simulink model "linearized_smm_with_lqr_2d"  (R2014b)
settings: Solver=FixedStepDiscrete  StartTime=0.0  StopTime=inf  FixedStep=sample_time  RelTol=1e-3
undefined symbols (not defined in the file): A_kalman_fourbar_gear, A_kalman_transverse, A_kalman_vertical, A_lpf_dtau, A_lpf_leg_spring, B1_lpf_dtau, B1_lpf_leg_spring, B2_lpf_dtau, B2_lpf_leg_spring, B_dx_versus_x0, B_kalman_fourbar_gear, B_kalman_transverse, B_kalman_vertical, backwards_K_sag_of_t, boom_mount_angle, C_kalman_fourbar_gear, C_kalman_transverse, C_kalman_vertical, com_leg_motor, com_torso, contact_threshold, control_start_time, d_vertical_boom_com_offset, d_vertical_com, desired_com_apex_height, desired_com_forward_velocity, desired_torso_angle, Discrete, fcut_contact, forward_dx, forward_dx_of_dxstar, forward_x, forward_x_of_dxstar, g, h_boom, HIP_MTR_MAX_CONT_TORQUE, i_robot, initial_dx_estimate, initial_dy_estimate, initial_dz_estimate, initial_z_estimate, j_leg, j_motor, j_segments, k_LQR_vertical, k_sea, k_vertical_winch, kalman_load_to_deflect_transmission, kalman_stance_slip_threshold, kd_lateral, kd_motor, kp_lateral, kp_motor, l_boom_projected, l_retract_delta, l_retract_swing_max, l_retract_swing_min, l_seg, lambda1, lambda2 ... (+60)
libraries: simulink x14, ctrlSharedLib x7
(part 4 of 4)

== matlab function linearized_smm_with_lqr_2d/Control/Behavior Control/Primary Leg Behavior/Running/Closed Loop Compensation/ESTIMATE CLOSED LOOP ERROR X FOR VARIABLE SPEED ==
  data: dx_land_hist input; A_cl output; delta_ux_hist input; dx_lift_hist input; dx_star_hist input; B_dx_versus_x0 parameter; W_real input; epsilon_0 output; c output; A_cl_nb output; epsilon_0_nb output; c_nb output
function [A_cl, epsilon_0, c, ...
          A_cl_nb, epsilon_0_nb, c_nb] = error_fitting_dxstar...
         (dx_land_hist, delta_ux_hist, dx_lift_hist, dx_star_hist,...
          B_dx_versus_x0, W_real)
% data_length = min([length(dx_lift_hist), filter_length]);
data_length = length(dx_lift_hist);
assert(data_length < 100);
% add fake data
fake_dx_land_err_magnitude = 0.1; fake_dx_star_magnitude = 0.1;
[fgrid_dx_land_err, fgrid_dx_star, fgrid_dx_lift_err] = ...
    meshgrid(fake_dx_land_err_magnitude*[-1 1],fake_dx_star_magnitude*[-1 1],0);
fake_data_length = numel(fgrid_dx_land_err);
fake_dx_land_err = fgrid_dx_land_err(:);
fake_dx_star = fgrid_dx_star(:);
fake_dx_lift_err = fgrid_dx_lift_err(:);
fake_delta_ux = zeros(fake_data_length,1);
% assert(fake_data_length<100);
% assert(filter_length<100);
% fake_dx_land_err = linspace(-0.1, 0.1, fake_data_length)';
% fake_dx_lift_err = zeros(fake_data_length,1);
% fake_delta_ux = zeros(fake_data_length,1);
% fake_dx_star = linspace(-0.25, 0.25, fake_data_length)';
dx_land_err = [reshape(dx_land_hist(1:data_length)-dx_star_hist(1:data_length),...
                       data_length, 1); fake_dx_land_err];
dx_lift_err = [reshape(dx_lift_hist(1:data_length)-dx_star_hist(1:data_length),...
                       data_length, 1); fake_dx_lift_err];
dx_star = [reshape(dx_star_hist(1:data_length), data_length,1); fake_dx_star];
delta_ux = [reshape(delta_ux_hist(1:data_length), data_length, 1); fake_delta_ux];
% weighted least squares
W = diag([W_real*ones(1,data_length), ones(1,fake_data_length)]);
Y = dx_lift_err - B_dx_versus_x0*delta_ux;
X = [dx_land_err, dx_star, ones(data_length+fake_data_length,1)];
% linear regression for s_{i+1}-s0 = A_cl*(s_i-s0) + epsilon_0 + c(s0) + B*delta_u
% solve for Y = X*beta, beta column vector
beta_hat = (X'*W*X)\X'*W*Y;
W_nobias = diag([W_real*ones(1,data_length), 0.001*ones(1,fake_data_length)]);
beta_hat_nobias = (X'*W_nobias*X)\X'*W_nobias*Y;
A_cl = beta_hat(1);
c = beta_hat(2);
epsilon_0 = beta_hat(3);
A_cl_nb = beta_hat_nobias(1);
c_nb = beta_hat_nobias(2);
epsilon_0_nb = beta_hat_nobias(3);

== matlab function linearized_smm_with_lqr_2d/Control/Behavior Control/Primary Leg Behavior/Running/Closed Loop Compensation/CLOSED LOOP COMPENSATION Y FOR VAIRABLE SPEED ==
  data: A_cl input; epsilon input; c input; delta_s_i input; dx_star input; B_cl input; delta_ux output
function delta_ux  = closed_loop_compensation_dxstar...
         (A_cl,epsilon, c, delta_s_i, dx_star, B_cl)
% assume form of delta_s_{i+1} = A_cl*delta_s_i + epsilon +c*dx_star + B_cl*delta_ux
% where delta measures deviation from deadbeat case. solve for
% delta_ux = (-A_cl*delta_s_i-epsilon - c*dxstar)/B_cl to achieve deadbeat
delta_ux = (-A_cl*delta_s_i - epsilon - c*dx_star)/B_cl;

== matlab function linearized_smm_with_lqr_2d/Control/Behavior Control/Primary Secondary Leg Swap/ToggleRightLeftLeg ==
  data: toggle input boolean; right_left output double; previous_right_left input double
function right_left = ToggleRightLeftLeg(toggle, previous_right_left)
    
    if toggle
        right_left = -previous_right_left + 1;
    else
        right_left = previous_right_left;
    end

end

== matlab function linearized_smm_with_lqr_2d/Control/Behavior Control/Lateral Control ==
  data: hopping input; right_left input; tau_r output size=1; qLateralR input; dqLateralR input; qLateralL input; dqLateralL input; F_leg_R input; F_leg_L input; deadbeat_enabled input; target_primary_deadbeat_angle input; lateral_transition_force parameter; lateral_target_angle_right parameter; m_leg_motor parameter; m_leg parameter; m_total_real parameter; g parameter; lateral_offset parameter; tau_l output size=1; kp_lateral parameter; kd_lateral parameter; minimum_lateral_angle parameter; maximum_lateral_angle parameter; HIP_MTR_MAX_CONT_TORQUE parameter; torso_centerline_roll_offset_angle parameter
function [tau_r, tau_l] = LateralBoomControl(hopping, right_left, qLateralR, dqLateralR, qLateralL, dqLateralL, F_leg_R, F_leg_L, deadbeat_enabled, target_primary_deadbeat_angle, lateral_transition_force, lateral_target_angle_right, m_leg_motor, m_leg, m_total_real, g, lateral_offset, kp_lateral, kd_lateral, minimum_lateral_angle, maximum_lateral_angle, HIP_MTR_MAX_CONT_TORQUE, torso_centerline_roll_offset_angle)
    
    % Only add gravity compensation to PD when suspended from winch (approximately static)
    gravity_compensation = 0;
    if ~hopping, gravity_compensation = (m_leg_motor+m_leg)*g*lateral_offset; end
    
    % Inertia for feedforward accelerations
    motor_inertia = (m_leg_motor+m_leg)*lateral_offset^2;
    
    % Right Leg
    right_target = [lateral_target_angle_right, 0, 0];
    if deadbeat_enabled && right_left
        right_target = [pi/2 - target_primary_deadbeat_angle(1) - torso_centerline_roll_offset_angle, -target_primary_deadbeat_angle(2), -target_primary_deadbeat_angle(2)];
    end
    desired = [saturate(right_target(1),minimum_lateral_angle,maximum_lateral_angle), right_target(2)];
    measured = [qLateralR, dqLateralR];
    tau_r = [kp_lateral, kd_lateral] * (desired-measured)' + gravity_compensation + motor_inertia*right_target(3);
    tau_r = max(min(HIP_MTR_MAX_CONT_TORQUE, tau_r),-HIP_MTR_MAX_CONT_TORQUE);
    
    if (F_leg_R >= lateral_transition_force)
        if hopping
            tau_r = -F_leg_R*lateral_offset*(m_total_real-(m_leg_motor+m_leg))/m_total_real;
        else
            tau_r = -lateral_offset*(F_leg_R-(m_leg_motor+m_leg)*g);
        end
    end
    
    % Left Leg
    left_target = [lateral_target_angle_right, 0, 0];
    if deadbeat_enabled && ~right_left
        left_target = [pi/2 - target_primary_deadbeat_angle(1) + torso_centerline_roll_offset_angle, -target_primary_deadbeat_angle(2), -target_primary_deadbeat_angle(2)];
    end
    desired = [saturate(left_target(1),minimum_lateral_angle,maximum_lateral_angle), left_target(2)];
    measured = [qLateralL, dqLateralL];
    tau_l = [kp_lateral, kd_lateral] * (desired-measured)' + gravity_compensation + motor_inertia*left_target(3);
    tau_l = max(min(HIP_MTR_MAX_CONT_TORQUE, tau_l),-HIP_MTR_MAX_CONT_TORQUE);
    
    if (F_leg_L >= lateral_transition_force)
        if hopping
            tau_l = -F_leg_L*lateral_offset*(m_total_real-(m_leg_motor+m_leg))/m_total_real;
        else
            tau_l = -lateral_offset*(F_leg_L-(m_leg_motor+m_leg)*g);
        end
    end
end

function [desired_saturated] = saturate(desired, minimum_lateral_angle, maximum_lateral_angle)
    desired_saturated = desired;
    if desired(1) < minimum_lateral_angle
        desired_saturated = [minimum_lateral_angle, 0];
    elseif desired(1) > maximum_lateral_angle
        desired_saturated = [maximum_lateral_angle, 0];    
    end
end

== matlab function linearized_smm_with_lqr_2d/Control/Behavior Control/Primary Leg Behavior/Running/Stance/Inverse Dynamics 2D/target_GRF_inverse_dynamics ==
  data: GRFx input; GRFz input; right_left input; z output; theta input; phi input; l_leg input; w input; tau_rotor_f input; tau_rotor_b input; d_vertical_com parameter; LEG_MTR_GEAR_RATIO parameter; g parameter; j_leg parameter; i_robot parameter; m_total_real parameter; m_leg parameter
%% Inverse dynamics
% Inputs:  gamma, dgamma, theta, dtheta,  GRFx_des, GRFy_des
% Outputs: ddx,   ddy,    ddl,   ddgamma, ddtheta,  tau_sf,  tau_sb
function z = fcn(GRFx, GRFz, right_left, theta, phi, l_leg, w,...
                                  tau_rotor_f, tau_rotor_b, ...
                                  d_vertical_com, LEG_MTR_GEAR_RATIO, g,...
                                  j_leg, i_robot, ...
                                  m_total_real, m_leg)

              
              
    % Parameters
    m      = m_total_real;    % mass of system + boom
    Il     = j_leg;             % inertia of leg
    It     = i_robot;           % inertia of system3.
    d      = d_vertical_com;             % distance from hip to system COM
    g1     = phi(1)+theta(1);   % global leg angle (after spring)
    dg1    = phi(2)+theta(2);
    th     = theta(1);          % global torso angle   
    dth    = theta(2);
    t_rf   = tau_rotor_f;       % torque applied at front rotor 
    t_rb   = tau_rotor_b;       % torque applied at back rotor
    N      = -LEG_MTR_GEAR_RATIO;
    l      = l_leg(1);          % leg length
    dl     = l_leg(2);
    
    % Stance dynamics (P z = [h; -dJ*dq] + [J zeros(2,2)]^T F)
    %     J  = [1  0  sin(g1)     l*cos(g1)   -d*cos(th);
    %           0  1  cos(g1)    -l*sin(g1)    d*sin(th)];
    %       
    %     dJ = [0  0   dg1*cos(g1)    (-l*dg1*sin(g1)+dl*cos(g1))  d*dth*sin(th);
    %           0  0  -dg1*sin(g1)    (-1*dg1*cos(g1)-dl*sin(g1))  d*dth*cos(th)];
    % 
    %     dq  = [dx  dz  dl  dg1  dth ]';
    %       
    %     M = [m  0   0       0    0; 
    %          0  m   0       0    0;
    %          0  0   m_leg   0    0;   
    %          0  0   0       Il   0;  
    %          0  0   0       0    It];  
    %     
    %     h = [0; -m*g_reduced; 0; 0; (-t_rf-t_rb)];
    % 
    %     S = [ 0         0;
    %           0         0;
    %           1/w      -1/w;
    %           1         1;
    %          -(N-1)/N  -(N-1)/N];
    % 
    %     F = [GRFx GRFz]';
    %     
    %     P = [M              -S;       
    %          J               zeros(2,2)];
    
    % Solving for z:    
    %     ddq = [ddx ddy ddl ddg1 ddth]';
    %     z = [ddq; t_sf; t_sb];
    %     z = P\([h; -dJ*dq] + [J zeros(2,2)]'*F);
    
    z =  [GRFx/m;
         (GRFz - g*m)/m;
        -(Il*d*dg1^2*m*cos(g1 - th) - 2*GRFx*Il*d*sin(th) - 2*Il*d^2*dth^2*m - GRFz*d*l^2*m*cos(th) - GRFx*d*l^2*m*sin(th) - 2*GRFz*Il*d*cos(th) + 2*GRFz*It*N*l*cos(g1) + 2*GRFz*Il*N*d*cos(th) + 2*GRFx*It*N*l*sin(g1) + 2*GRFx*Il*N*d*sin(th) - It*N*dg1^2*l*m + GRFz*d*l^2*m*cos(2*g1 - th) + GRFx*d*l^2*m*sin(2*g1 - th) + 2*Il*d*g*m*cos(th) + Il*d*dg1^2*m*cos(g1 + th) + 2*Il*N*d^2*dth^2*m - It*N*dg1^2*l^2*m - 2*It*N*g*l*m*cos(g1) - 2*Il*N*d*g*m*cos(th) + It*N*dg1^2*l^2*m*cos(2*g1) - Il*N*d*dg1^2*m*cos(g1 + th) - Il*d*dg1^2*l*m*cos(g1 + th) + 4*Il*d*dg1*dl*m*sin(g1 - th) + GRFz*N*d^2*l*m*cos(g1) + GRFz*N*d*l^2*m*cos(th) + GRFx*N*d^2*l*m*sin(g1) + 2*N*d*l*m*t_rb*sin(g1 - th) + 2*N*d*l*m*t_rf*sin(g1 - th) + GRFx*N*d*l^2*m*sin(th) - Il*N*d*dg1^2*m*cos(g1 - th) - GRFz*N*d^2*l*m*cos(g1 - 2*th) + GRFx*N*d^2*l*m*sin(g1 - 2*th) + Il*d*dg1^2*l*m*cos(g1 - th) - It*N*dg1^2*l*m*cos(2*g1) - GRFz*N*d*l^2*m*cos(2*g1 - th) - GRFx*N*d*l^2*m*sin(2*g1 - th) + Il*N*d*dg1^2*l*m*cos(g1 + th) - 4*Il*N*d*dg1*dl*m*sin(g1 - th) - Il*N*d*dg1^2*l*m*cos(g1 - th) + 2*It*N*d*dth^2*l*m*cos(g1 - th))/(2*m*(It*N*l - Il*d*cos(g1 - th) + Il*N*d*cos(g1 - th)));
        -(2*GRFx*It*N*cos(g1) - 2*GRFz*It*N*sin(g1) + GRFx*N*d^2*m*cos(g1 - 2*th) + 4*It*N*dg1*dl*m + GRFz*N*d^2*m*sin(g1 - 2*th) + GRFx*d*l*m*cos(2*g1 - th) - GRFz*d*l*m*sin(2*g1 - th) + It*N*dg1^2*m*sin(2*g1) + 2*It*N*g*m*sin(g1) + GRFx*d*l*m*cos(th) - GRFz*d*l*m*sin(th) + GRFx*N*d^2*m*cos(g1) + 2*N*d*m*t_rb*cos(g1 - th) + 2*N*d*m*t_rf*cos(g1 - th) - GRFz*N*d^2*m*sin(g1) - GRFx*N*d*l*m*cos(th) + GRFz*N*d*l*m*sin(th) - GRFx*N*d*l*m*cos(2*g1 - th) - 2*It*N*d*dth^2*m*sin(g1 - th) + GRFz*N*d*l*m*sin(2*g1 - th) - It*N*dg1^2*l*m*sin(2*g1))/(2*m*(It*N*l - Il*d*cos(g1 - th) + Il*N*d*cos(g1 - th)));
        -(GRFx*Il*cos(g1) - GRFz*Il*sin(g1) - GRFx*Il*N*cos(g1) + (Il*dg1^2*m*sin(2*g1))/2 + GRFz*Il*N*sin(g1) + Il*g*m*sin(g1) + GRFx*l^2*m*cos(g1) - GRFz*l^2*m*sin(g1) + 2*Il*dg1*dl*m + N*l*m*t_rb + N*l*m*t_rf + GRFz*N*l^2*m*sin(g1) - 2*Il*N*dg1*dl*m - Il*d*dth^2*m*sin(g1 - th) - (Il*N*dg1^2*m*sin(2*g1))/2 - (Il*dg1^2*l*m*sin(2*g1))/2 - Il*N*g*m*sin(g1) - GRFx*N*l^2*m*cos(g1) + GRFx*N*d*l*m*cos(th) - GRFz*N*d*l*m*sin(th) + Il*N*d*dth^2*m*sin(g1 - th) + (Il*N*dg1^2*l*m*sin(2*g1))/2)/(m*(It*N*l - Il*d*cos(g1 - th) + Il*N*d*cos(g1 - th)));
        -(2*GRFx*Il*It*N*cos(g1) - 2*GRFz*Il*It*N*sin(g1) - GRFz*Il*d*m*w*cos(th) - 2*GRFz*Il*d*m_leg*w*cos(th) - GRFx*Il*d*m*w*sin(th) - 2*GRFx*Il*d*m_leg*w*sin(th) + GRFx*Il*N*d^2*m*cos(g1) + 2*Il*N*d*m*t_rb*cos(g1 - th) + 2*Il*N*d*m*t_rf*cos(g1 - th) + 2*GRFx*It*N*l^2*m*cos(g1) - GRFz*Il*N*d^2*m*sin(g1) - 2*GRFz*It*N*l^2*m*sin(g1) + GRFx*Il*N*d^2*m*cos(g1 - 2*th) + 4*Il*It*N*dg1*dl*m + GRFz*Il*N*d^2*m*sin(g1 - 2*th) - 2*Il*d^2*dth^2*m*m_leg*w - GRFz*Il*d*m*w*cos(2*g1 - th) - GRFx*Il*d*m*w*sin(2*g1 - th) + Il*It*N*dg1^2*m*sin(2*g1) + 2*Il*It*N*g*m*sin(g1) - GRFx*d*l^2*m*m_leg*w*sin(th) - Il*It*N*dg1^2*l*m*sin(2*g1) + Il*d*dg1^2*m*m_leg*w*cos(g1 - th) + 2*GRFz*It*N*l*m*w*cos(g1) + 2*GRFz*It*N*l*m_leg*w*cos(g1) + GRFz*Il*N*d*m*w*cos(th) + 2*GRFz*Il*N*d*m_leg*w*cos(th) + 2*GRFx*It*N*l*m*w*sin(g1) + 2*GRFx*It*N*l*m_leg*w*sin(g1) + GRFx*Il*N*d*m*w*sin(th) + 2*GRFx*Il*N*d*m_leg*w*sin(th) - It*N*dg1^2*l*m*m_leg*w + GRFz*d*l^2*m*m_leg*w*cos(2*g1 - th) + GRFx*d*l^2*m*m_leg*w*sin(2*g1 - th) + 2*Il*d*g*m*m_leg*w*cos(th) + Il*d*dg1^2*m*m_leg*w*cos(g1 + th) + 2*Il*N*d^2*dth^2*m*m_leg*w - It*N*dg1^2*l^2*m*m_leg*w - 2*Il*It*N*d*dth^2*m*sin(g1 - th) + GRFz*Il*N*d*m*w*cos(2*g1 - th) + GRFx*Il*N*d*m*w*sin(2*g1 - th) - GRFz*d*l^2*m*m_leg*w*cos(th) + It*N*dg1^2*l^2*m*m_leg*w*cos(2*g1) - Il*N*d*dg1^2*m*m_leg*w*cos(g1 + th) - Il*d*dg1^2*l*m*m_leg*w*cos(g1 + th) + 4*Il*d*dg1*dl*m*m_leg*w*sin(g1 - th) + GRFz*N*d^2*l*m*m_leg*w*cos(g1) + GRFz*N*d*l^2*m*m_leg*w*cos(th) + GRFx*N*d^2*l*m*m_leg*w*sin(g1) + 2*N*d*l*m*m_leg*t_rb*w*sin(g1 - th) + 2*N*d*l*m*m_leg*t_rf*w*sin(g1 - th) + GRFx*N*d*l^2*m*m_leg*w*sin(th) - Il*N*d*dg1^2*m*m_leg*w*cos(g1 - th) - GRFz*N*d^2*l*m*m_leg*w*cos(g1 - 2*th) + GRFx*N*d^2*l*m*m_leg*w*sin(g1 - 2*th) + Il*d*dg1^2*l*m*m_leg*w*cos(g1 - th) - It*N*dg1^2*l*m*m_leg*w*cos(2*g1) - GRFz*N*d*l^2*m*m_leg*w*cos(2*g1 - th) - GRFx*N*d*l^2*m*m_leg*w*sin(2*g1 - th) - 2*It*N*g*l*m*m_leg*w*cos(g1) - 2*Il*N*d*g*m*m_leg*w*cos(th) + Il*N*d*dg1^2*l*m*m_leg*w*cos(g1 + th) - 4*Il*N*d*dg1*dl*m*m_leg*w*sin(g1 - th) - Il*N*d*dg1^2*l*m*m_leg*w*cos(g1 - th) + 2*It*N*d*dth^2*l*m*m_leg*w*cos(g1 - th))/(4*m*(It*N*l - Il*d*cos(g1 - th) + Il*N*d*cos(g1 - th)));
         (2*GRFz*Il*It*N*sin(g1) - 2*GRFx*Il*It*N*cos(g1) - GRFz*Il*d*m*w*cos(th) - 2*GRFz*Il*d*m_leg*w*cos(th) - GRFx*Il*d*m*w*sin(th) - 2*GRFx*Il*d*m_leg*w*sin(th) - GRFx*Il*N*d^2*m*cos(g1) - 2*Il*N*d*m*t_rb*cos(g1 - th) - 2*Il*N*d*m*t_rf*cos(g1 - th) - 2*GRFx*It*N*l^2*m*cos(g1) + GRFz*Il*N*d^2*m*sin(g1) + 2*GRFz*It*N*l^2*m*sin(g1) - GRFx*Il*N*d^2*m*cos(g1 - 2*th) - 4*Il*It*N*dg1*dl*m - GRFz*Il*N*d^2*m*sin(g1 - 2*th) - 2*Il*d^2*dth^2*m*m_leg*w - GRFz*Il*d*m*w*cos(2*g1 - th) - GRFx*Il*d*m*w*sin(2*g1 - th) - Il*It*N*dg1^2*m*sin(2*g1) - 2*Il*It*N*g*m*sin(g1) - GRFx*d*l^2*m*m_leg*w*sin(th) + Il*It*N*dg1^2*l*m*sin(2*g1) + Il*d*dg1^2*m*m_leg*w*cos(g1 - th) + 2*GRFz*It*N*l*m*w*cos(g1) + 2*GRFz*It*N*l*m_leg*w*cos(g1) + GRFz*Il*N*d*m*w*cos(th) + 2*GRFz*Il*N*d*m_leg*w*cos(th) + 2*GRFx*It*N*l*m*w*sin(g1) + 2*GRFx*It*N*l*m_leg*w*sin(g1) + GRFx*Il*N*d*m*w*sin(th) + 2*GRFx*Il*N*d*m_leg*w*sin(th) - It*N*dg1^2*l*m*m_leg*w + GRFz*d*l^2*m*m_leg*w*cos(2*g1 - th) + GRFx*d*l^2*m*m_leg*w*sin(2*g1 - th) + 2*Il*d*g*m*m_leg*w*cos(th) + Il*d*dg1^2*m*m_leg*w*cos(g1 + th) + 2*Il*N*d^2*dth^2*m*m_leg*w - It*N*dg1^2*l^2*m*m_leg*w + 2*Il*It*N*d*dth^2*m*sin(g1 - th) + GRFz*Il*N*d*m*w*cos(2*g1 - th) + GRFx*Il*N*d*m*w*sin(2*g1 - th) - GRFz*d*l^2*m*m_leg*w*cos(th) + It*N*dg1^2*l^2*m*m_leg*w*cos(2*g1) - Il*N*d*dg1^2*m*m_leg*w*cos(g1 + th) - Il*d*dg1^2*l*m*m_leg*w*cos(g1 + th) + 4*Il*d*dg1*dl*m*m_leg*w*sin(g1 - th) + GRFz*N*d^2*l*m*m_leg*w*cos(g1) + GRFz*N*d*l^2*m*m_leg*w*cos(th) + GRFx*N*d^2*l*m*m_leg*w*sin(g1) + 2*N*d*l*m*m_leg*t_rb*w*sin(g1 - th) + 2*N*d*l*m*m_leg*t_rf*w*sin(g1 - th) + GRFx*N*d*l^2*m*m_leg*w*sin(th) - Il*N*d*dg1^2*m*m_leg*w*cos(g1 - th) - GRFz*N*d^2*l*m*m_leg*w*cos(g1 - 2*th) + GRFx*N*d^2*l*m*m_leg*w*sin(g1 - 2*th) + Il*d*dg1^2*l*m*m_leg*w*cos(g1 - th) - It*N*dg1^2*l*m*m_leg*w*cos(2*g1) - GRFz*N*d*l^2*m*m_leg*w*cos(2*g1 - th) - GRFx*N*d*l^2*m*m_leg*w*sin(2*g1 - th) - 2*It*N*g*l*m*m_leg*w*cos(g1) - 2*Il*N*d*g*m*m_leg*w*cos(th) + Il*N*d*dg1^2*l*m*m_leg*w*cos(g1 + th) - 4*Il*N*d*dg1*dl*m*m_leg*w*sin(g1 - th) - Il*N*d*dg1^2*l*m*m_leg*w*cos(g1 - th) + 2*It*N*d*dth^2*l*m*m_leg*w*cos(g1 - th))/(4*m*(It*N*l - Il*d*cos(g1 - th) + Il*N*d*cos(g1 - th)))];


end

== matlab function linearized_smm_with_lqr_2d/Control/Behavior Control/Primary Leg Behavior/Running/Flight/Avoid Hitting Mechanical Limits ==
  data: back_cmd output double; front_cmd output double; dback_cmd output double; dfront_cmd output double; ddback_cmd output double; ddfront_cmd output double; back_desired input; dback_desired input; ddback_desired input; front_desired input; dfront_desired input; ddfront_desired input; min_front_bar_angle parameter; max_front_bar_angle parameter; min_back_bar_angle parameter; max_back_bar_angle parameter
%% Avoid joint limits by ensuring we don't command velocities/accelerations that would push us into them when we are close to them.
function [back_cmd, front_cmd, dback_cmd, dfront_cmd, ddback_cmd, ddfront_cmd] ...
    = AvoidFourbarLimits(back_desired,dback_desired, ddback_desired, ...
          front_desired, dfront_desired, ddfront_desired, ...
          min_front_bar_angle, max_front_bar_angle, min_back_bar_angle, max_back_bar_angle)
    [back_cmd, front_cmd, dback_cmd, dfront_cmd, ddback_cmd, ddfront_cmd] = AvoidFourbarLimits(back_desired,dback_desired, ddback_desired, front_desired, dfront_desired, ddfront_desired, min_front_bar_angle, max_front_bar_angle, min_back_bar_angle, max_back_bar_angle);
end

== matlab function linearized_smm_with_lqr_2d/Control/Behavior Control/Primary Leg Behavior/Running/Flight/Virtual Leg to Four Bar ==
  data: l_leg input; dl_leg input; ddl_leg input; phi input; dphi input; ddphi input; back output; dback output; ddback output; front output; dfront output; ddfront output
function [back, dback, ddback, front, dfront, ddfront] = VirtualLegToFourBar(l_leg, dl_leg, ddl_leg, phi, dphi, ddphi)
    [back, dback, ddback, front, dfront, ddfront] = VirtualLegToFourBar(l_leg, dl_leg, ddl_leg, phi, dphi, ddphi);
end

== matlab function linearized_smm_with_lqr_2d/Control/Behavior Control/Secondary Leg Behavior/Mirrored Leg Length Target ==
  data: primary_l_leg input; l_leg output; dl_leg output; primary_dl_leg input; l_retract_swing_min parameter; l_retract_swing_max parameter; ddl_leg output; l_retract_delta parameter
function [l_leg, dl_leg, ddl_leg] = LegLengthTarget(primary_l_leg, primary_dl_leg, l_retract_swing_min, l_retract_swing_max, l_retract_delta)

    l_leg = primary_l_leg - l_retract_delta;
    dl_leg = 0;
    ddl_leg = 0;
    if l_leg > l_retract_swing_min && l_leg < l_retract_swing_max
        dl_leg = primary_dl_leg;
    else
        l_leg = max(min(l_leg, l_retract_swing_max), l_retract_swing_min);
    end

end

== matlab function linearized_smm_with_lqr_2d/Control/Behavior Control/State Estimation/PositionUsingBoomEncoders ==
  data: horizontal_com_position output; qRoll input; dqRoll input; qYaw input; horizontal_com_velocity output; vertical_com_position output; dqYaw input; qPitch input; dqPitch input; l_boom_projected parameter; h_boom parameter; boom_mount_angle parameter; d_vertical_boom_com_offset parameter; vertical_com_velocity output; lateral_com_position output; lateral_com_velocity output
function [horizontal_com_position, horizontal_com_velocity, ...
          vertical_com_position, vertical_com_velocity, ...
          lateral_com_position, lateral_com_velocity ] = ...
         PositionUsingBoomEncoders(qRoll, dqRoll, qYaw, dqYaw, qPitch, dqPitch, ...
                        l_boom_projected, h_boom, boom_mount_angle, ...
                        d_vertical_boom_com_offset)
    
    % com position / velocity
    [ horizontal_com_position, horizontal_com_velocity, vertical_com_position, vertical_com_velocity, lateral_com_position, lateral_com_velocity ] = ComCalculationFromBoom( qRoll, dqRoll, qYaw, dqYaw, qPitch, dqPitch, l_boom_projected, h_boom, boom_mount_angle, d_vertical_boom_com_offset );
    
end

== matlab function linearized_smm_with_lqr_2d/Fourbar Gearside Kalman Filter/External Trunk Torque Estimate ==
  data: grf_xz input; rotor_torque input; spring_torque input; tau_trunk output; torso_pitch input; d_vertical_com parameter; LEG_MTR_GEAR_RATIO parameter
function tau_trunk = tau_trunk(grf_xz, rotor_torque, spring_torque, torso_pitch, d_vertical_com, LEG_MTR_GEAR_RATIO )
    d = d_vertical_com;
    theta = torso_pitch;
    N = LEG_MTR_GEAR_RATIO;
    tau_trunk = sum(-rotor_torque + -(N-1)/N*spring_torque) + (-d*cos(theta)*grf_xz(1) + d*sin(theta)*grf_xz(2));
end

== matlab function linearized_smm_with_lqr_2d/Fourbar Gearside Kalman Filter/Covariance Estimates ==
  data: spring_torque input; absolute_gear input; current_position_estimate input; state_uncertainty input; Q1 output; R1 output; Q2 output; R2 output; R_kalman_absolute_normal parameter; R_kalman_absolute_fail parameter; R_kalman_incremental_unloaded parameter; R_kalman_incremental_loaded parameter; kalman_load_to_deflect_transmission parameter; Q3 output; R3 output; Q4 output; R4 output; max_absolute_measurement_innovation parameter; k_sea parameter; Q_kalman_spring_torque parameter; Q_kalman_rotor_torque parameter; Q_kalman_trunk_torque parameter; sample_time parameter
function [Q1, R1, Q2, R2, Q3, R3, Q4, R4] = covariance( spring_torque, absolute_gear, current_position_estimate, state_uncertainty, R_kalman_absolute_normal, R_kalman_absolute_fail, R_kalman_incremental_unloaded, R_kalman_incremental_loaded, kalman_load_to_deflect_transmission, max_absolute_measurement_innovation, k_sea, Q_kalman_spring_torque, Q_kalman_rotor_torque, Q_kalman_trunk_torque, sample_time)

    persistent previous_absolute_gear
    if isempty(previous_absolute_gear)
        previous_absolute_gear = absolute_gear;
    end
    
    % Measurement covariance
    R_absolute = ones(4,1)*R_kalman_absolute_normal;
    dropped_out = previous_absolute_gear == absolute_gear;
    out_of_range = abs(current_position_estimate - absolute_gear) > max_absolute_measurement_innovation;
    R_absolute(dropped_out | out_of_range) = R_kalman_absolute_fail;
    
    R_incremental_scale = min(abs(spring_torque)/kalman_load_to_deflect_transmission, 1);
    R_incremental = R_incremental_scale*R_kalman_incremental_loaded + (1-R_incremental_scale)*R_kalman_incremental_unloaded;
    
    R1 = diag([R_absolute(1), R_incremental(1)])/sample_time;
    R2 = diag([R_absolute(2), R_incremental(2)])/sample_time;
    R3 = diag([R_absolute(3), R_incremental(3)])/sample_time;
    R4 = diag([R_absolute(4), R_incremental(4)])/sample_time;
    
    % Process noise covariance
    Q_spring_torque = k_sea'.^2.*(state_uncertainty + R_kalman_absolute_normal) + Q_kalman_spring_torque;

    Q1 = diag([Q_spring_torque(1), Q_kalman_rotor_torque, Q_kalman_trunk_torque]);
    Q2 = diag([Q_spring_torque(2), Q_kalman_rotor_torque, Q_kalman_trunk_torque]);
    Q3 = diag([Q_spring_torque(3), Q_kalman_rotor_torque, Q_kalman_trunk_torque]);
    Q4 = diag([Q_spring_torque(4), Q_kalman_rotor_torque, Q_kalman_trunk_torque]);

    previous_absolute_gear = absolute_gear;
end

== matlab function linearized_smm_with_lqr_2d/Fourbar Gearside Kalman Filter/eigen values 1 ==
  data: Z input; E output
function E = eigen(Z)
    E = real(eig(Z));
    E = sort(E);
end

== matlab function linearized_smm_with_lqr_2d/Fourbar Gearside Kalman Filter/eigen values 2 ==
  data: Z input; E output
function E = eigen(Z)
    E = real(eig(Z));
    E = sort(E);
end

== matlab function linearized_smm_with_lqr_2d/Fourbar Gearside Kalman Filter/eigen values 3 ==
  data: Z input; E output
function E = eigen(Z)
    E = real(eig(Z));
    E = sort(E);
end

== matlab function linearized_smm_with_lqr_2d/Fourbar Gearside Kalman Filter/eigen values4  ==
  data: Z input; E output
function E = eigen(Z)
    E = real(eig(Z));
    E = sort(E);
end

== matlab function linearized_smm_with_lqr_2d/Control/Behavior Control/Primary Leg Behavior/Running/Flight/Avoid Virtual Leg Length Limits ==
  data: l_leg_desired input; dl_leg_desired input; ddl_leg_desired input; l_leg_cmd output double; dl_leg_cmd output double; ddl_leg_cmd output double; min_leg_length parameter; max_leg_length parameter
%% Avoid virtual leg length limits by ensuring we don't command position/velocities/accelerations that would hit them.
function [l_leg_cmd, dl_leg_cmd, ddl_leg_cmd] = AvoidVirtualLengthLimits(l_leg_desired, dl_leg_desired, ddl_leg_desired, min_leg_length, max_leg_length)
    [l_leg_cmd, dl_leg_cmd, ddl_leg_cmd] = AvoidVirtualLengthLimits(l_leg_desired, dl_leg_desired, ddl_leg_desired, min_leg_length, max_leg_length);
end

== matlab function linearized_smm_with_lqr_2d/Control/Behavior Control/Primary Leg Behavior/Running/Flight/Calculate Time Until Touchdown ==
  data: z_dz input; t output; z_land parameter; g parameter
function t = EstimateTouchdown(z_dz, z_land, g)
  z_hat = z_dz(1); 
  dz_hat = z_dz(2);
  t = (-dz_hat-sqrt( max(dz_hat^2 - 4*g/2*(z_land-z_hat),0) ))/(-g);
end

== matlab function linearized_smm_with_lqr_2d/Control/Behavior Control/Primary Leg Behavior/Running/Closed Loop Compensation/ESTIMATE CLOSED LOOP ERROR Y FOR VARIABLE SPEED ==
  data: dx_land_hist input; A_cl output; delta_ux_hist input; dx_lift_hist input; dx_star_hist input; B_dx_versus_x0 parameter; W_real input; epsilon_0 output; c output; A_cl_nb output; epsilon_0_nb output; c_nb output
function [A_cl, epsilon_0, c, ...
          A_cl_nb, epsilon_0_nb, c_nb] = error_fitting_dxstar...
         (dx_land_hist, delta_ux_hist, dx_lift_hist, dx_star_hist,...
          B_dx_versus_x0, W_real)
% data_length = min([length(dx_lift_hist), filter_length]);
data_length = length(dx_lift_hist);
assert(data_length < 100);
% add fake data
fake_dx_land_err_magnitude = 0.1; fake_dx_star_magnitude = 0.1;
[fgrid_dx_land_err, fgrid_dx_star, fgrid_dx_lift_err] = ...
    meshgrid(fake_dx_land_err_magnitude*[-1 1],fake_dx_star_magnitude*[-1 1],0);
fake_data_length = numel(fgrid_dx_land_err);
fake_dx_land_err = fgrid_dx_land_err(:);
fake_dx_star = fgrid_dx_star(:);
fake_dx_lift_err = fgrid_dx_lift_err(:);
fake_delta_ux = zeros(fake_data_length,1);
% assert(fake_data_length<100);
% assert(filter_length<100);
% fake_dx_land_err = linspace(-0.1, 0.1, fake_data_length)';
% fake_dx_lift_err = zeros(fake_data_length,1);
% fake_delta_ux = zeros(fake_data_length,1);
% fake_dx_star = linspace(-0.25, 0.25, fake_data_length)';
dx_land_err = [reshape(dx_land_hist(1:data_length)-dx_star_hist(1:data_length),...
                       data_length, 1); fake_dx_land_err];
dx_lift_err = [reshape(dx_lift_hist(1:data_length)-dx_star_hist(1:data_length),...
                       data_length, 1); fake_dx_lift_err];
dx_star = [reshape(dx_star_hist(1:data_length), data_length,1); fake_dx_star];
delta_ux = [reshape(delta_ux_hist(1:data_length), data_length, 1); fake_delta_ux];
% weighted least squares
W = diag([W_real*ones(1,data_length), ones(1,fake_data_length)]);
Y = dx_lift_err - B_dx_versus_x0*delta_ux;
X = [dx_land_err, dx_star, ones(data_length+fake_data_length,1)];
% linear regression for s_{i+1}-s0 = A_cl*(s_i-s0) + epsilon_0 + c(s0) + B*delta_u
% solve for Y = X*beta, beta column vector
beta_hat = (X'*W*X)\X'*W*Y;
W_nobias = diag([W_real*ones(1,data_length), 0.001*ones(1,fake_data_length)]);
beta_hat_nobias = (X'*W_nobias*X)\X'*W_nobias*Y;
A_cl = beta_hat(1);
c = beta_hat(2);
epsilon_0 = beta_hat(3);
A_cl_nb = beta_hat_nobias(1);
c_nb = beta_hat_nobias(2);
epsilon_0_nb = beta_hat_nobias(3);

== matlab function linearized_smm_with_lqr_2d/Control/Behavior Control/Primary Leg Behavior/Running/Circular Buffer/Buffer ==
  data: data input; buffer output size=recorded_steps; trigger input; buffer_size input
function buffer  = buffer_data(data, trigger, buffer_size)

    persistent buffer_memory
    coder.varsize('buffer_memory',100);
    if isempty(buffer_memory)
        buffer_memory = [];
    end
    
    if trigger
        buffer_memory = [data; buffer_memory];
        if size(buffer_memory, 1) > buffer_size
            buffer_memory = buffer_memory(1:buffer_size,:);
        end
    end
    
    buffer = buffer_memory;

end

== matlab function linearized_smm_with_lqr_2d/Control/Behavior Control/Primary Leg Behavior/Running/Circular Buffer/Buffer1 ==
  data: data input; buffer output size=recorded_steps; trigger input; buffer_size input
function buffer  = buffer_data(data, trigger, buffer_size)

    persistent buffer_memory
    coder.varsize('buffer_memory',100);
    if isempty(buffer_memory)
        buffer_memory = [];
    end
    
    if trigger
        buffer_memory = [data; buffer_memory];
        if size(buffer_memory, 1) > buffer_size
            buffer_memory = buffer_memory(1:buffer_size,:);
        end
    end
    
    buffer = buffer_memory;

end

== matlab function linearized_smm_with_lqr_2d/Control/Behavior Control/Primary Leg Behavior/Running/Circular Buffer/Buffer2 ==
  data: data input; buffer output size=recorded_steps; trigger input; buffer_size input
function buffer  = buffer_data(data, trigger, buffer_size)

    persistent buffer_memory
    coder.varsize('buffer_memory',100);
    if isempty(buffer_memory)
        buffer_memory = [];
    end
    
    if trigger
        buffer_memory = [data; buffer_memory];
        if size(buffer_memory, 1) > buffer_size
            buffer_memory = buffer_memory(1:buffer_size,:);
        end
    end
    
    buffer = buffer_memory;

end

== matlab function linearized_smm_with_lqr_2d/Control/Behavior Control/Primary Leg Behavior/Running/Circular Buffer/Buffer3 ==
  data: data input; buffer output size=recorded_steps; trigger input; buffer_size input
function buffer  = buffer_data(data, trigger, buffer_size)

    persistent buffer_memory
    coder.varsize('buffer_memory',100);
    if isempty(buffer_memory)
        buffer_memory = [];
    end
    
    if trigger
        buffer_memory = [data; buffer_memory];
        if size(buffer_memory, 1) > buffer_size
            buffer_memory = buffer_memory(1:buffer_size,:);
        end
    end
    
    buffer = buffer_memory;

end

== matlab function linearized_smm_with_lqr_2d/Control/Behavior Control/Primary Leg Behavior/Running/Circular Buffer/Buffer4 ==
  data: data input; buffer output size=recorded_steps; trigger input; buffer_size input
function buffer  = buffer_data(data, trigger, buffer_size)

    persistent buffer_memory
    coder.varsize('buffer_memory',100);
    if isempty(buffer_memory)
        buffer_memory = [];
    end
    
    if trigger
        buffer_memory = [data; buffer_memory];
        if size(buffer_memory, 1) > buffer_size
            buffer_memory = buffer_memory(1:buffer_size,:);
        end
    end
    
    buffer = buffer_memory;

end

== matlab function linearized_smm_with_lqr_2d/Control/Behavior Control/Primary Leg Behavior/Running/Circular Buffer/Buffer5 ==
  data: data input; buffer output size=recorded_steps; trigger input; buffer_size input
function buffer  = buffer_data(data, trigger, buffer_size)

    persistent buffer_memory
    coder.varsize('buffer_memory',100);
    if isempty(buffer_memory)
        buffer_memory = [];
    end
    
    if trigger
        buffer_memory = [data; buffer_memory];
        if size(buffer_memory, 1) > buffer_size
            buffer_memory = buffer_memory(1:buffer_size,:);
        end
    end
    
    buffer = buffer_memory;

end

== matlab function linearized_smm_with_lqr_2d/Control/Behavior Control/State Estimation/Kalman Filtering/Measurement Noise Covariance Matricies ==
  data: R_transverse output; vertical_GRF_L input; vertical_GRF_R input; R_kalman_foot_stance parameter; R_kalman_foot_slip parameter; R_kalman_dfoot_stance parameter; R_kalman_dfoot_slip parameter; sample_time parameter; m_total_real parameter; g parameter; R_vertical output; kalman_stance_slip_threshold parameter
function [R_transverse, R_vertical] =...
         MeasurementNoiseCovariance(vertical_GRF_L, vertical_GRF_R, ...
           R_kalman_foot_stance, R_kalman_foot_slip, R_kalman_dfoot_stance, R_kalman_dfoot_slip, sample_time, m_total_real, g, kalman_stance_slip_threshold)

    % filter states: [dx_w]; [dy_w]; [dz_w];
    % measurements:  [dx_w-dfL + dfL_hat; dx_w-dfR + dfR_hat]; 

    ratio_L = max(0, min(vertical_GRF_L/(kalman_stance_slip_threshold*m_total_real*g),1)); % ratio is 0 if no load, 1 if at least equilibrium
    ratio_R = max(0, min(vertical_GRF_R/(kalman_stance_slip_threshold*m_total_real*g),1));
    R_transverse = diag([ratio_L*R_kalman_dfoot_stance + (1-ratio_L)*R_kalman_dfoot_slip, ...
                         ratio_R*R_kalman_dfoot_stance + (1-ratio_R)*R_kalman_dfoot_slip])/sample_time;
    R_vertical = diag([ratio_L*R_kalman_foot_stance  + (1-ratio_L)*R_kalman_foot_slip,...
                       ratio_L*R_kalman_dfoot_stance + (1-ratio_L)*R_kalman_dfoot_slip,...
                       ratio_R*R_kalman_foot_stance  + (1-ratio_R)*R_kalman_foot_slip,...
                       ratio_R*R_kalman_dfoot_stance + (1-ratio_R)*R_kalman_dfoot_slip])/sample_time;
end
